simulink model "widePosSysWithContr"  (R2018a)
settings: Solver=VariableStepAuto  StartTime=0.0  StopTime=10.0  RelTol=1e-3
values from neighbouring files (symbols this model uses):
  Kd = K*T    [Untitled2.m]    (also in modelParam.m; widePosSysAnal.m)
  Kp = K*Zc/Pc    [Untitled2.m]    (also in modelParam.m; widePosSysAnal.m)
undefined symbols (not defined in the file or in its folder): gpden, gpnum
settings Model: Creator=tumma  LastModifiedBy=tumma
settings SolverCC: ZeroCrossAlgorithm=Adaptive
settings DebuggingCC: MaxConsecutiveZCsMsg=none

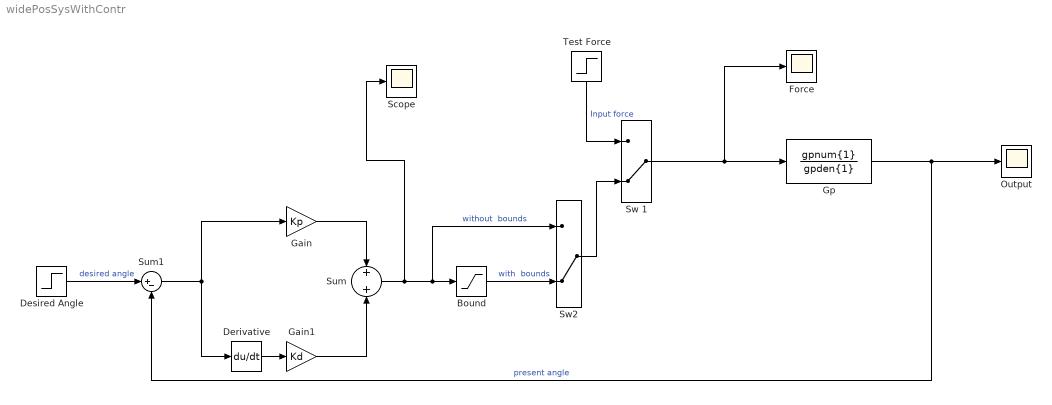
== system widePosSysWithContr ==
  "Bound " : Saturate  UpperLimit=0.411  LowerLimit=-0.411
  Derivative : Derivative
  "Desired Angle " : Step  After=5  SampleTime=0
  Force : Scope
  Gain : Gain  Gain=Kp
  Gain1 : Gain  Gain=Kd
  Gp : TransferFcn  Numerator=gpnum{1}  Denominator=gpden{1}
  "Output " : Scope
  Scope : Scope
  Sum : Sum
  Sum1 : Sum  Inputs=|+-
  "Sw 1 " : ManualSwitch  CurrentSetting=0
  "Sw2 " : ManualSwitch  CurrentSetting=0
  Test Force : Step  After=0.0901  SampleTime=0
  wires:
  "Bound "/1 -> "Sw2 "/2  "with  bounds"
  Sum/1 -> Scope/1, "Sw2 "/1, "Bound "/1  "without  bounds"
  Sum1/1 -> Gain/1, Derivative/1
  "Sw2 "/1 -> "Sw 1 "/2
  "Desired Angle "/1 -> Sum1/1  "desired angle"
  Derivative/1 -> Gain1/1
  "Sw 1 "/1 -> Force/1, Gp/1
  Gain/1 -> Sum/1
  Test Force/1 -> "Sw 1 "/1  "Input force"
  Gain1/1 -> Sum/2
  Gp/1 -> Sum1/2, "Output "/1  "present angle"
